simulink library "winch000_cl"  (R2018b)
settings: Solver=VariableStepAuto  StartTime=0.0  StopTime=10.0  RelTol=1e-3
undefined symbols (not defined in the file): winch
libraries: firstOrderFilter_ul x1
settings Model: Creator=mcobb  LastModifiedBy=mcobb

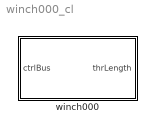
== system winch000_cl ==
  winch000 : Subsystem

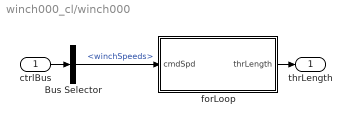
== system winch000_cl/winch000 ==
  ctrlBus : Inport  OutDataTypeStr=Bus: ctrlBus
  Bus Selector : BusSelector  OutputSignals=winchSpeeds
  forLoop : Subsystem  mask{wnch=winch}
      mask prompts: wnch "Winch Structure"
  thrLength : Outport
  wires:
  forLoop/1(thrLength) -> thrLength/1
  ctrlBus/1 -> Bus Selector/1
  Bus Selector/1 -> forLoop/1(cmdSpd)  "<winchSpeeds>"

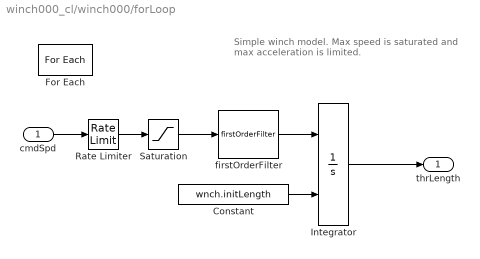
== system winch000_cl/winch000/forLoop ==
  note: Simple winch model.  Max speed is saturated
      | and max acceleration is limited.
  cmdSpd : Inport  Partition=on  PartitionDimension=1  PartitionWidth=1  PartitionOffset=0
  Constant : Constant  Value=wnch.initLength
  For Each : ForEach  DisableCoverage=on  IterateSubsysMaskParameter=on  SubsysMaskParameterIterationDimension=2  IndexMode=One-based
  Integrator : Integrator  InitialConditionSource=external
  Rate Limiter : RateLimiter  RisingSlewLimit=wnch.maxAccel  FallingSlewLimit=-wnch.maxAccel  SampleTimeMode=inherited
  Saturation : Saturate  UpperLimit=wnch.maxSpeed  LowerLimit=-wnch.maxSpeed  LinearizeAsGain=off
  firstOrderFilter : firstOrderFilter_ul/firstOrderFilter  tau=wnch.timeConst  ic=0
  thrLength : Outport  ConcatenationDimension=1
  wires:
  cmdSpd/1 -> Rate Limiter/1
  Integrator/1 -> thrLength/1
  Constant/1 -> Integrator/2
  Rate Limiter/1 -> Saturation/1
  Saturation/1 -> firstOrderFilter/1
  firstOrderFilter/1 -> Integrator/1
